simulink model "Simulacion_Diagrama_Electrico_VE"  (R2016a)
settings: Solver=VariableStepAuto  StartTime=0.0  StopTime=1.2  RelTol=1e-3
undefined symbols (not defined in the file or in its folder): A, B, C
settings Model: Creator=Daniel  LastModifiedBy=Daniel

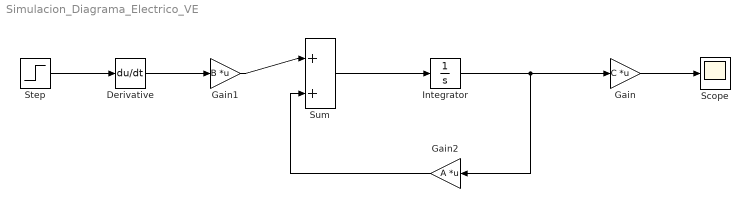
== system Simulacion_Diagrama_Electrico_VE ==
  Derivative : Derivative
  Gain : Gain  Gain=C  Multiplication=Matrix(K*u) (u vector)
  Gain1 : Gain  Gain=B  Multiplication=Matrix(K*u) (u vector)
  Gain2 : Gain  Gain=A  Multiplication=Matrix(K*u) (u vector)
  Integrator : Integrator
  Scope : Scope
  Step : Step  After=2  SampleTime=0
  Sum : Sum  Inputs=|++
  wires:
  Gain1/1 -> Sum/1
  Sum/1 -> Integrator/1
  Integrator/1 -> Gain2/1, Gain/1
  Gain2/1 -> Sum/2
  Gain/1 -> Scope/1
  Step/1 -> Derivative/1
  Derivative/1 -> Gain1/1
